simulink model "ControlModel2_PID_NoFAN_NoBJT_Commented"  (R2022b)
settings: Solver=VariableStepAuto  StartTime=0.0  StopTime=600.0  RelTol=1e-3
libraries: simulink x1
settings Model: Creator=damia  LastModifiedBy=enric
settings DebuggingCC: UnconnectedInputMsg=warning  UnconnectedOutputMsg=warning  UnconnectedLineMsg=warning
settings ModelReferenceCC: EnableRefExpFcnMdlSchedulingChecks=on
settings RTWCC: DLArmComputeVersion=19.05

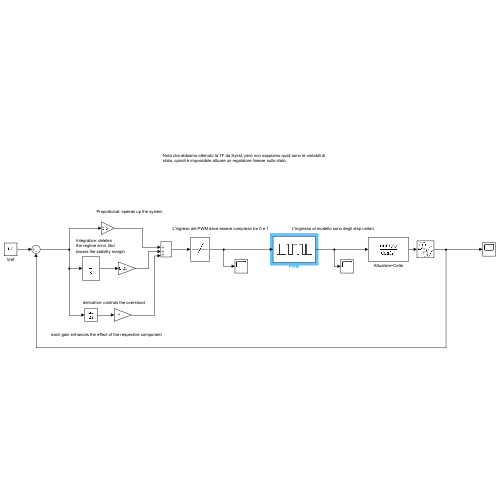
[thumbnail: Simulink's stored preview of the top-level diagram]
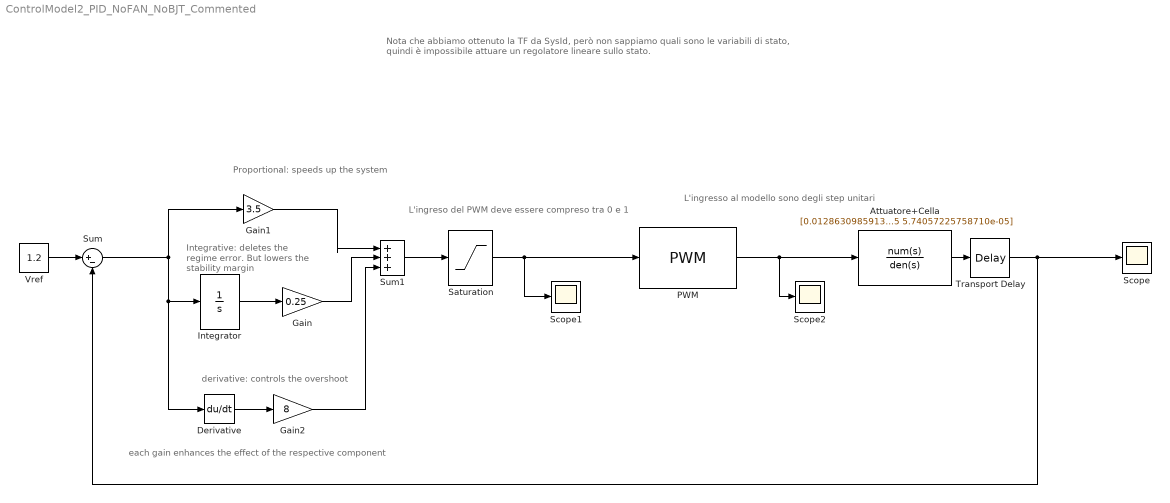
== system ControlModel2_PID_NoFAN_NoBJT_Commented ==
  note: each gain enhances the effect of the respective component
  note: derivative: controls the overshoot
  note: Integrative: deletes
      | the regime error. But
      | lowers the stability margin
  note: Proportional: speeds up the system
  note: Nota che abbiamo ottenuto la TF da SysId, però non sappiamo quali sono le variabili di stato, quindi è impossibile attuare un regolatore lineare sullo stato.
  note: L'ingreso del PWM deve essere compreso tra 0 e 1
  note: L'ingresso al modello sono degli step unitari
  Attuatore+Cella : TransferFcn  Numerator=[0.0128630985913695 9.75217482279844e-05]  Denominator=[1 0.278653761544147 0.0104105852135155 5.74057225758710e-05]
  Derivative : Derivative
  Gain : Gain  Gain=0.25
  Gain1 : Gain  Gain=3.5
  Gain2 : Gain  Gain=8
  Integrator : Integrator  UpperSaturationLimit=0
  PWM : simulink/Discontinuities/PWM  DisableCoverage=on  Period=0.002  InitialDelay=0  DisallowZeroDutyCycle=off  RunAtFixedTimeIntervals=off  SampleTime=0.1
  Saturation : Saturate  UpperLimit=1  LowerLimit=0
  Scope : Scope
  Scope1 : Scope
  Scope2 : Scope
  Sum : Sum  Inputs=|+-
  Sum1 : Sum  Inputs=|+++
  Transport Delay : TransportDelay
  Vref : Constant  Value=1.2
  wires:
  PWM/1 -> Scope2/1, Attuatore+Cella/1
  Saturation/1 -> Scope1/1, PWM/1
  Integrator/1 -> Gain/1
  Gain/1 -> Sum1/2
  Attuatore+Cella/1 -> Transport Delay/1
  Sum/1 -> Gain1/1, Derivative/1, Integrator/1
  Vref/1 -> Sum/1
  Transport Delay/1 -> Scope/1, Sum/2
  Gain1/1 -> Sum1/1
  Sum1/1 -> Saturation/1
  Derivative/1 -> Gain2/1
  Gain2/1 -> Sum1/3
